simulink model "c_lab2sim"  (R2020b)
settings: Solver=FixedStepAuto  StartTime=0.0  StopTime=10.0  FixedStep=0.001  RelTol=1e-3
libraries: dspsrcs4 x1
settings Model: Creator=musa oğural  LastModifiedBy=musa oğural

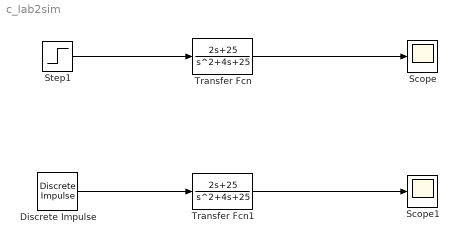
== system c_lab2sim ==
  Discrete Impulse : dspsrcs4/Discrete  Impulse  Delay=0  SampleTime=1  FrameSample=1  OutputFrames=off  dataType=double  isSigned=on  wordLen=16  udDataType=sfix(16)  fracBitsMode=Best precision  numFracBits=15  OutDataTypeStr=double  LastOutDataTypeStr=double
  Scope : Scope
  Scope1 : Scope
  Step1 : Step  Time=0  SampleTime=0
  Transfer Fcn : TransferFcn  Numerator=[2 25]  Denominator=[1 4 25]
  Transfer Fcn1 : TransferFcn  Numerator=[2 25]  Denominator=[1 4 25]
  wires:
  Step1/1 -> Transfer Fcn/1
  Transfer Fcn/1 -> Scope/1
  Discrete Impulse/1 -> Transfer Fcn1/1
  Transfer Fcn1/1 -> Scope1/1
